simulink subsystem "s0323_mechanical_simulator2"  (R2019b)
settings: Solver=VariableStepAuto  StartTime=0.0  StopTime=10.0  RelTol=1e-3
model mask{th_0=0, al_0=0, th_dot_0=0, al_dot_0=0}
  mask prompts: th_0 "Initial theta"; al_0 "Initial alpha"; th_dot_0 "Initial theta dot"; al_dot_0 "Initial alpha dot"
undefined symbols (not defined in the file): PARAMS
settings Model: Creator=paolo  LastModifiedBy=alessandro
settings DebuggingCC: SFMachineParentedDataDiag=error

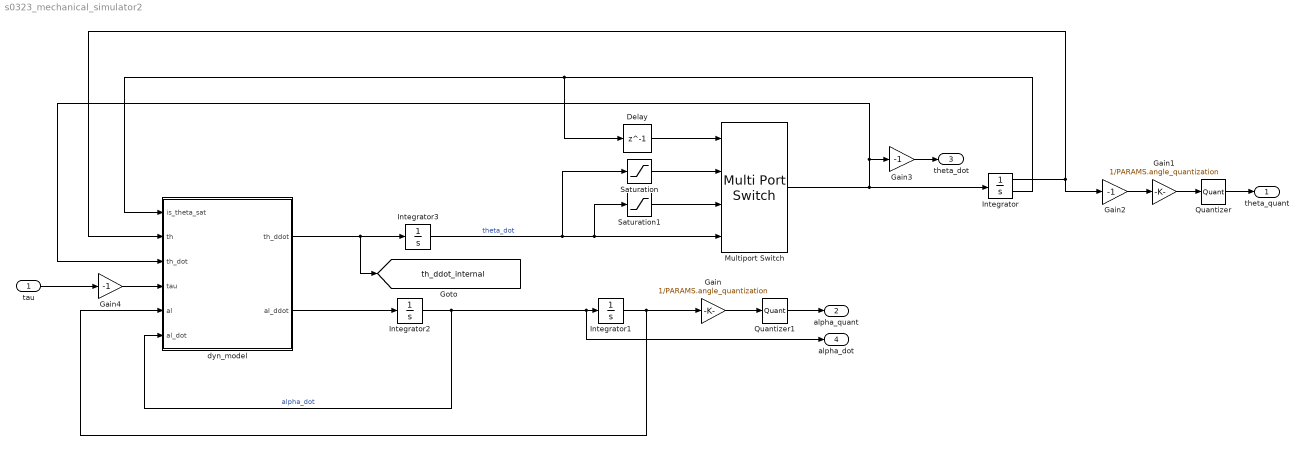
== system s0323_mechanical_simulator2 ==
  tau : Inport  Unit=N*m  PortDimensions=1
  Delay : Delay  DelayLength=1
  Gain : Gain  Gain=1/PARAMS.angle_quantization
  Gain1 : Gain  Gain=1/PARAMS.angle_quantization
  Gain2 : Gain  Gain=-1
  Gain3 : Gain  Gain=-1
  Gain4 : Gain  Gain=-1
  Integrator : Integrator  InitialCondition=th_0  LimitOutput=on  UpperSaturationLimit=135/180*pi  LowerSaturationLimit=-135/180*pi  ShowSaturationPort=on
  Integrator1 : Integrator  InitialCondition=al_0  UpperSaturationLimit=0.01  LowerSaturationLimit=-0.01
  Integrator2 : Integrator  InitialCondition=al_dot_0  UpperSaturationLimit=0.01  LowerSaturationLimit=-0.01
  Integrator3 : Integrator  InitialCondition=th_dot_0  UpperSaturationLimit=0.001  LowerSaturationLimit=-0.001
  Multiport Switch : MultiPortSwitch  DataPortOrder=Specify indices  DataPortIndices={-1,1,0}
  Quantizer : Quantizer  QuantizationInterval=1
  Quantizer1 : Quantizer  QuantizationInterval=1
  Saturation : Saturate  UpperLimit=inf  LowerLimit=0
  Saturation1 : Saturate  UpperLimit=0  LowerLimit=-inf
  dyn_model : MATLAB Function  TreatAsAtomicUnit=on
  theta_quant : Outport  Unit=rad  PortDimensions=1
  alpha_quant : Outport  Port=2  Unit=rad  PortDimensions=1
  theta_dot : Outport  Port=3  Unit=rad/s  PortDimensions=1
  alpha_dot : Outport  Port=4  Unit=rad/s  PortDimensions=1
  tag scope: th_ddot_internal=global
  wires:
  Integrator1/1 -> dyn_model/5(al), Gain/1
  Integrator2/1 -> dyn_model/6(al_dot), Integrator1/1, alpha_dot/1  "alpha_dot"
  Integrator3/1 -> Multiport Switch/4, Saturation1/1, Saturation/1  "theta_dot"
  dyn_model/1(th_ddot) -> Integrator3/1, [th_ddot_internal]
  dyn_model/2(al_ddot) -> Integrator2/1
  tau/1 -> Gain4/1
  Integrator/1 -> dyn_model/2(th), Gain2/1
  Quantizer/1 -> theta_quant/1
  Integrator/2 -> dyn_model/1(is_theta_sat), Delay/1
  Multiport Switch/1 -> Gain3/1, dyn_model/3(th_dot), Integrator/1
  Delay/1 -> Multiport Switch/1
  Saturation/1 -> Multiport Switch/2
  Saturation1/1 -> Multiport Switch/3
  Quantizer1/1 -> alpha_quant/1
  Gain/1 -> Quantizer1/1
  Gain1/1 -> Quantizer/1
  Gain2/1 -> Gain1/1
  Gain3/1 -> theta_dot/1
  Gain4/1 -> dyn_model/4(tau)

== matlab function s0323_mechanical_simulator2/dyn_model ==
  data: is_theta_sat input; th input; th_dot input size=1; tau input size=1; th_ddot output; al input size=1; al_dot input size=1; al_ddot output size=1; PARAMS parameter
function [th_ddot, al_ddot] = dyn_model(is_theta_sat, th, th_dot, tau, al, al_dot, PARAMS)

    m2 = PARAMS.mp;
    L2 = PARAMS.Lp;
    m1 = PARAMS.mr;
    L1 = PARAMS.Lr;
    Jm = PARAMS.Jm;
    Jh = PARAMS.Jh;
    Cth = PARAMS.Cth;
    Cal = PARAMS.Cal;
    Dth = PARAMS.Dth;
    K = PARAMS.K;
    Sth = PARAMS.Sth;
    th_0 = PARAMS.th_0_cable;
    
    if is_theta_sat == 1 % theta clamped at 135 deg
        if tau > K*(th-th_0)
            tau = K*(th-th_0);
        end
    elseif is_theta_sat == -1 % theta clamped at -135 deg
        if tau < K*(th-th_0)
            tau = K*(th-th_0);
        end
    end

    if abs(th_dot) < PARAMS.Sth_vel_threshold
        if abs(tau - K*(th-th_0)) < Sth
            tau_static_friction = tau - K*(th-th_0);
        else
            tau_static_friction = Sth;
        end
        tau_dynamic_friction = 0;
    else
        tau_static_friction = 0;
        tau_dynamic_friction = Dth*sign(th_dot);
    end
    
    tau_actual = tau - tau_static_friction - tau_dynamic_friction;
    g = 9.81;
    
    th_ddot = -(12*Cth*L2*th_dot - sin(al)*(6*L1*m2*L2^2*al_dot^2 + 9*L1*g*m2*cos(al)*L2) - 12*L2*tau_actual + 12*K*L2*th - 12*K*L2*th_0 - 18*Cal*L1*al_dot*cos(al) + 4*L2^3*al_dot*m2*th_dot*sin(2*al) + 3*L1*L2^2*m2*th_dot^2*sin(2*al)*cos(al))/(L2*(12*Jh + 12*Jm + 4*L1^2*m1 + 12*L1^2*m2 - 9*L1^2*m2*cos(al)^2 + 4*L2^2*m2*sin(al)^2));
    al_ddot = -(36*Cal*Jh*al_dot + 36*Cal*Jm*al_dot + 12*Cal*L1^2*al_dot*m1 + 36*Cal*L1^2*al_dot*m2 + 6*L2^3*g*m2^2*sin(al)^3 + 12*Cal*L2^2*al_dot*m2*sin(al)^2 + 18*L1^2*L2*g*m2^2*sin(al) + (9*L1^2*L2^2*al_dot^2*m2^2*sin(2*al))/2 - 6*L1^2*L2^2*m2^2*th_dot^2*sin(2*al) + 18*L1*L2*m2*tau_actual*cos(al) + 18*Jh*L2*g*m2*sin(al) + 18*Jm*L2*g*m2*sin(al) - 4*L2^4*m2^2*th_dot^2*cos(al)*sin(al)^3 - 6*Jh*L2^2*m2*th_dot^2*sin(2*al) - 6*Jm*L2^2*m2*th_dot^2*sin(2*al) + 6*L1^2*L2*g*m1*m2*sin(al) - 2*L1^2*L2^2*m1*m2*th_dot^2*sin(2*al) - 18*Cth*L1*L2*m2*th_dot*cos(al) - 18*K*L1*L2*m2*th*cos(al) + 18*K*L1*L2*m2*th_0*cos(al) + 12*L1*L2^3*al_dot*m2^2*th_dot*sin(al)*(sin(al)^2 - 1))/(L2^2*m2*(12*Jh + 12*Jm + 4*L1^2*m1 + 3*L1^2*m2 + 9*L1^2*m2*sin(al)^2 + 4*L2^2*m2*sin(al)^2));
 
    
end
